simulink model "OpAmpWithNoise"  (R2024a)
settings: Solver=VariableStepAuto  StartTime=0.0  StopTime=1e-4  MaxStep=1e-5  RelTol=1e-3  EnableMultiTasking=on
PreLoadFcn:
  | bw = 2*pi*10e6; % 10MHz bandwidth
  | R2 = 1e6;
  | R1 = 1e4;
  | C1 = 1/(R2*bw);
  | ts = 1e-8; % Simulation step size
libraries: ee_lib x5, fl_lib x5, nesl_utility x2
CloseFcn:
  | try,close(h1_OpAmpWithNoise),end
  | clear h1_OpAmpWithNoise
  | try,close(h2_OpAmpWithNoise),end
  | clear h2_OpAmpWithNoise
  | try,close(h3_OpAmpWithNoise),end
  | clear h3_OpAmpWithNoise
  | try,close(h4_OpAmpWithNoise),end
  | clear h4_OpAmpWithNoise
  | 
  | 
  | clear simlog_OpAmpWithNoise
  | clear logsout_OpAmpWithNoise
  | clear C1 R1 R2 bw ts
Description:
  | Op-Amp with Noise
settings Model: Creator=The MathWorks, Inc.  LastModifiedBy=The MathWorks, Inc.
settings SolverCC: AlgebraicLoopSolver=TrustRegion
settings DataIOCC: LimitDataPoints=on  MaxDataPoints=195000  SaveFormat=Array  ReturnWorkspaceOutputs=off  SignalLoggingName=logsout_OpAmpWithNoise
settings OptimizationCC: ReuseModelBlockBuffer=off  ExpressionDepthLimit=2147483647  LifeSpan=inf
settings DebuggingCC: UnderspecifiedInitializationDetection=Classic  MergeDetectMultiDrivingBlocksExec=none  UnconnectedInputMsg=warning  UnconnectedOutputMsg=warning  UnconnectedLineMsg=warning  StateNameClashWarn=warning  SFUnexpectedBacktrackingDiag=warning  SFNoUnconditionalDefaultTransitionDiag=warning  SFExecutionAtInitializationDiag=none  ArithmeticOperatorsInVariantConditions=warning
settings HardwareCC: ProdBitPerPointer=32  ProdBitPerSizeT=32  ProdBitPerPtrDiffT=32  ProdLargestAtomicFloat=None  ProdIntDivRoundTo=Undefined  ProdEndianess=Unspecified  ProdWordSize=32  ProdHWDeviceType=32-bit Generic
settings ModelReferenceCC: EnableRefExpFcnMdlSchedulingChecks=on  PropagateSignalLabelsOutOfModel=off
settings SFSimCC: SimUseLocalCustomCode=off  CustomCodeUndefinedFunction=UseInterfaceOnly
settings RTWCC: RTWUseLocalCustomCode=off  GPUComputeCapability=3.5  DLArmComputeVersion=19.05
settings CodeAppCC: StateflowObjectComments=on
settings GRTTargetCC: TargetLangStandard=C89/C90 (ANSI)
settings ConfigComp: CovMetricSettings=dw  CovSaveCumulativeToWorkspaceVar=on  CovSaveSingleToWorkspaceVar=on  CovExternalEMLEnable=off  CovSFcnEnable=off
settings SimscapeCC: SimscapeLogType=all  SimscapeLogSimulationStatistics=on  SimscapeLogName=simlog_OpAmpWithNoise  SimscapeLogDataHistory=195000

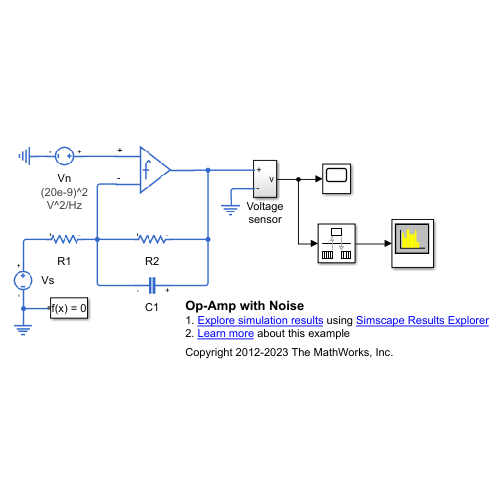
[thumbnail: Simulink's stored preview of the top-level diagram]
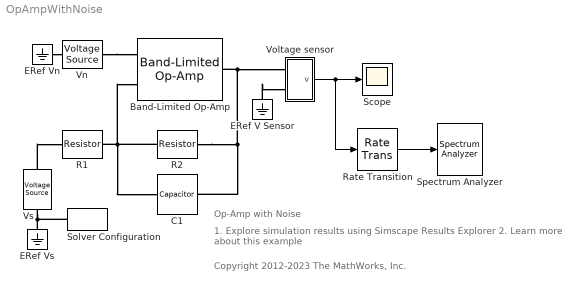
== system OpAmpWithNoise ==
  note: Op-Amp with Noise
  note: 1. Explore simulation results using Simscape Results Explorer
      | 2. Learn more about this example
  note: Copyright 2012-2023 The MathWorks, Inc.
  " R1 " : ee_lib/Passive/Resistor  R=R1 Ohm  enable_R_tol=0  R_tol=5  tol_distribution=1  nSigma=4  enable_operating_limits=0  operating_limit_action=2  power_rating=1 W  max_working_voltage=100 V  enable_faults=ee.enum.enable.no  fault_action=simscape.enum.assert.action.none  R_faulted=Inf Ohm  fault_trigger=ee.enum.faults.faultTrigger.temporal  t_fault=1 s  max_permissible_current=1 A  t_fail_on_current=1 s  noise_mode=0  Tdevice=25 degC  sample_time=ts s  repeatability=1  user_seed=0  auto_seed=622576118  faulted_specify=off  faulted_priority=None  faulted=0  power_derating_T1=70 degC  power_derating_T2=155 degC  operating_temperature_range_vec=[-50, 150] degC  alpha=3.93e-3 1/K  Tmeas=25 degC  thermal_mass=100 J/K  temperature_specify=off  temperature_priority=High  temperature=298.15 K  temperature_nominal_specify=off  temperature_nominal_value=1  temperature_nominal_unit=K
  Band-Limited Op-Amp : ee_lib/Integrated Circuits/Band-Limited Op-Amp  A=1e5  Rin=10 MOhm  Rout=100 Ohm  Vmin=-15 V  Vmax=15 V  Vdotmax=1e10 V/s  f=10 MHz  V0=0 V
  C1 : fl_lib/Electrical/Electrical Elements/Capacitor  c=C1 F  r=1e-6 Ohm  g=0 1/Ohm  i_specify=off  i_priority=High  i=0 A  i_nominal_specify=off  i_nominal_value=1  i_nominal_unit=A  v_specify=off  v_priority=High  v=0 V  v_nominal_specify=off  v_nominal_value=1  v_nominal_unit=V  vc_specify=on  vc_priority=High  vc=0 V  vc_nominal_specify=off  vc_nominal_value=1  vc_nominal_unit=V
  ERef V Sensor : fl_lib/Electrical/Electrical Elements/Electrical Reference
  ERef Vn : fl_lib/Electrical/Electrical Elements/Electrical Reference
  ERef Vs : fl_lib/Electrical/Electrical Elements/Electrical Reference
  R2 : ee_lib/Passive/Resistor  R=R2 Ohm  enable_R_tol=0  R_tol=5  tol_distribution=1  nSigma=4  enable_operating_limits=0  operating_limit_action=2  power_rating=1 W  max_working_voltage=100 V  enable_faults=ee.enum.enable.no  fault_action=simscape.enum.assert.action.none  R_faulted=Inf Ohm  fault_trigger=ee.enum.faults.faultTrigger.temporal  t_fault=1 s  max_permissible_current=1 A  t_fail_on_current=1 s  noise_mode=0  Tdevice=25 degC  sample_time=ts s  repeatability=1  user_seed=0  auto_seed=51119000  faulted_specify=off  faulted_priority=None  faulted=0  power_derating_T1=70 degC  power_derating_T2=155 degC  operating_temperature_range_vec=[-50, 150] degC  alpha=3.93e-3 1/K  Tmeas=25 degC  thermal_mass=100 J/K  temperature_specify=off  temperature_priority=High  temperature=298.15 K  temperature_nominal_specify=off  temperature_nominal_value=1  temperature_nominal_unit=K
  Rate Transition : RateTransition  OutPortSampleTime=ts
  Scope : Scope
  Solver Configuration : nesl_utility/Solver Configuration  PhysicalDomain=network_engine_domain  SubClassName=solver  LeftPortType=input  RightPortType=generic  Tones=[]  Harmonics=[]  SimulateNoise=off  Profile=off  UseLocalSampling=off  EnableSwitchedLinearOptims=on  FrequencyDomain=off  UseCCode=off  RelTol=0.001  AbsTol=1e-06  MinStep=1e-09  ToWorkspace=off  RevertToSquareIcSolve=off  NumHomotopyIterations=100  PhasorMode=off  PhasorModeNumHarmonics=1  ConsistencySolver=NEWTON_FTOL  IndexReductionMethod=DerivativeReplacement  DoDC=off  ResidualTolerance=1e-9  ConsistencyTolSource=GLOBAL  ConsistencyAbsTol=0.001  ConsistencyRelTol=0.001  ConsistencyTolFactor=0.001  UseLocalSolver=off  LocalSolverChoice=NE_TRAPEZOIDAL_ADVANCER  ResolveIndetEquations=on  FunctionEvalNumThread=1  LocalSolverSampleTime=ts  DoFixedCost=off  MaxNonlinIter=3  MaxModeIter=2  ComputeImpulses=off  ImpulseIterations=2  LinearAlgebra=auto  LinearAlgebraNumThread=0  EquationFormulation=NE_TIME_EF  DelaysMemoryBudget=1024  AutomaticFiltering=on  FilteringTimeConstant=0.001  PartitionStorageMethod=AS_NEEDED  PartitionMemoryBudget=1024  PartitionMethod=FAST  MultibodyUseLocalSolver=off  MultibodyLocalSolverChoice=ODE1  MultibodyLocalSolverSampleTime=0.001
  Spectrum Analyzer : SpectrumAnalyzer  Tag=PublishSpectrum  WindowPosition=[544.2 454.6 483.2 324]  SpectrumType=Power density  Method=Welch  SampleRate=100000000  PlotAsTwoSidedSpectrum=off  RBWSource=Property  RBW=293e3  Span=50000000  CenterFrequency=25000000  StartFrequency=0  StopFrequency=50000000  AveragingMethod=Running  SpectrumUnits=dBm/Hz  YLabel=dBm / Hz  YLimits=[-131.91103900660184,-19.685082878216345]  ShowGrid=off  AllowFFTLengthLessThanSamplesPerUpdate=on
  Vn : ee_lib/Sources/Voltage Source  dc_voltage=0 V  ac_voltage=0 V  ac_shift=0 deg  ac_frequency=10 MHz  noise_mode=1  PSD=(20e-9)^2 V^2/Hz  sample_time=ts s  repeatability=1  user_seed=0  auto_seed=3890346746  i_specify=off  i_priority=None  i=0 A  i_nominal_specify=off  i_nominal_value=1  i_nominal_unit=A  v_specify=off  v_priority=None  v=0 V  v_nominal_specify=off  v_nominal_value=1  v_nominal_unit=V
      settings: AttributesFormatString=|
      | %<PSD>
      | %<PSD_unit>
  Voltage sensor : Subsystem
      settings: CopyFcn=set_param(gcb,'LinkStatus','none')
  Vs : ee_lib/Sources/Voltage Source  dc_voltage=0 V  ac_voltage=0.01 V  ac_shift=0 deg  ac_frequency=10 MHz  noise_mode=0  PSD=0 V^2/Hz  sample_time=0.001 s  repeatability=1  user_seed=0  auto_seed=2349385303  i_specify=off  i_priority=None  i=0 A  i_nominal_specify=off  i_nominal_value=1  i_nominal_unit=A  v_specify=off  v_priority=None  v=0 V  v_nominal_specify=off  v_nominal_value=1  v_nominal_unit=V
  wires:
  Voltage sensor/1(v) -> Rate Transition/1, Scope/1
  Rate Transition/1 -> Spectrum Analyzer/1
  connections:
  R2/LConn1 -- Band-Limited Op-Amp/LConn2 -- C1/RConn1 -- " R1 "/RConn1
  R2/RConn1 -- C1/LConn1 -- Voltage sensor/LConn1 -- Band-Limited Op-Amp/RConn1
  ERef V Sensor/LConn1 -- Voltage sensor/LConn2
  ERef Vs/LConn1 -- Solver Configuration/RConn1 -- Vs/RConn1
  Vn/LConn1 -- Band-Limited Op-Amp/LConn1
  Vs/LConn1 -- " R1 "/LConn1
  ERef Vn/LConn1 -- Vn/RConn1

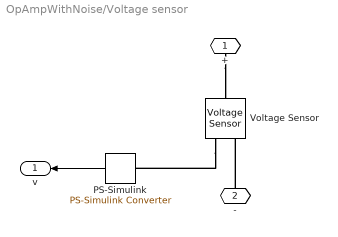
== system OpAmpWithNoise/Voltage sensor ==
  PS-Simulink : nesl_utility/PS-Simulink Converter  PhysicalDomain=network_engine_domain  SubClassName=ps_output  LeftPortType=input  RightPortType=output  PseudoPeriodic=off  Frequencies=[]  VectorFormat=1-D array  Unit=V  AffineConversion=off
  Voltage Sensor : fl_lib/Electrical/Electrical Sensors/Voltage Sensor
  + : PMIOPort  Side=Left
  - : PMIOPort  Port=2  Side=Left
  v : Outport  VectorParamsAs1DForOutWhenUnconnected=off
  wires:
  PS-Simulink/1 -> v/1
  connections:
  -/RConn1 -- Voltage Sensor/RConn2
  +/RConn1 -- Voltage Sensor/LConn1
  Voltage Sensor/RConn1 -- PS-Simulink/LConn1
